simulink model "VanDerPol"  (R2015b)
settings: Solver=ode4  StartTime=0.0  StopTime=30  FixedStep=0.01  RelTol=1e-3
InitFcn:
  | clear all; close all; clc;
  | mu=1;
  | x0=1;
  | xdot0=0;
  | StartTime=0;
  | EndTime=26.7;
  | 
  | % Design LQR for NO feedforward
  | A=[1 -1;1 0]; B=[-1;0]; C=[0 1]; D=[0]; Q=[1 0;0 1];  R=[1]
  | [K,S,E] = lqr(A,B,Q,R)
  | 
  | Kp=K(1);  Kd=K(2);  Ki=Kp*0.1;
  | Kpo=1;  Kdo=Kpo*1;  Kio=Kpo*0;
StopFcn:
  | figure(1);
  | subplot(3,1,1); plot(t,Trajectory(:,1),'--r','linewidth',3); grid; ylabel('x(t)','fontsize',16); title('Position, Rate, Acceleration Trajectories','fontsize',16);
  | hold on; plot(t,State(:,1),'linewidth',2); hold off; legend('Desired', 'Actual');
  | subplot(3,1,2); plot(t,Trajectory(:,2),'--r','linewidth',3);  grid; ylabel('xdot(t)','fontsize',16);
  | hold on; plot(t,State(:,2),'linewidth',2);  hold off; legend('Desired', 'Actual');
  | subplot(3,1,3); plot(t,Trajectory(:,3),'--r','linewidth',3);  grid; ylabel('xddot(t)','fontsize',16); xlabel('time (sec)','fontsize',16);
  | hold on; plot(t,State(:,3),'linewidth',2);  hold off; legend('Desired', 'Actual');
  | 
  | MeanErrorX=num2str(mean(Trajectory(:,1)-State(:,1))); MeanErrorXdot=num2str(mean(Trajectory(:,2)-State(:,2)));MeanErrorXddot=num2str(mean(Trajectory(:,1)-State(:,3)));
  | STDErrorX=num2str(std(Trajectory(:,1)-State(:,1))); STDErrorXdot=num2str(std(Trajectory(:,2)-State(:,2)));STDErrorXddot=num2str(std(Trajectory(:,1)-State(:,3)));
  | ErrorLabelX=['\mu =',MeanErrorX, ',  \sigma= ',STDErrorX];  ErrorLabelXdot=['\mu =',MeanErrorXdot, ',  \sigma= ',STDErrorXdot];  ErrorLabelXddot=['\mu =',MeanErrorXddot, ',  \sigma= ',STDErrorXddot];
  | 
  | figure(2)
  | subplot(3,1,1); plot(t,Trajectory(:,1)-State(:,1),'linewidth',2); axis tight; grid; ylabel('\delta_x_(_t_)','fontsize',16);
  | title('ERROR: Position, Rate, Acceleration Trajectories','fontsize',16);   legend(ErrorLabelX);
  | 
  | subplot(3,1,2); plot(t,Trajectory(:,2)-State(:,2),'linewidth',2); axis tight; grid; ylabel('\delta_x_d_o_t_(_t_)','fontsize',16);
  | legend(ErrorLabelXdot);
  | 
  | subplot(3,1,3); plot(t,Trajectory(:,3)-State(:,3),'linewidth',2); axis tight; grid; ylabel('\delta_x_d_d_o_t_(_t_)','fontsize',16);
  | xlabel('time (sec)','fontsize',16);  legend(ErrorLabelXddot);
  | 
  | figure(3)
  | subplot(2,1,1); plot(t,LuenbergerEstimationError(:,1),'linewidth',2); axis tight; grid; ylabel('Luenberger','fontsize',16); title('Estimation \delta_x_(_t_) Error','fontsize',16);
  | subplot(2,1,2); plot(t,PIDoEstimationError,'linewidth',2); axis tight; grid; ylabel('PID','fontsize',16);
  | 
  | figure(4);plot(State(:,1), State(:,2)); axis equal; grid;
  | xlabel('x(t)','fontsize',16);; ylabel('dx(t)/dt','fontsize',16); title('Phase Portrait','fontsize',16);
libraries: simulink_need_slupdate x1, simulink x1
settings Model: Creator=tsands  LastModifiedBy=tasands
settings DataIOCC: SaveFormat=Array
settings DebuggingCC: UnderspecifiedInitializationDetection=Classic  MergeDetectMultiDrivingBlocksExec=none  SolverPrmCheckMsg=warning
settings HardwareCC: ProdBitPerPointer=32  ProdLargestAtomicFloat=None  ProdIntDivRoundTo=Undefined  ProdEndianess=Unspecified  ProdWordSize=32  ProdHWDeviceType=32-bit Generic
settings GRTTargetCC: GeneratePreprocessorConditionals=Disable all
settings ConfigComp: CovModelRefEnable=Off

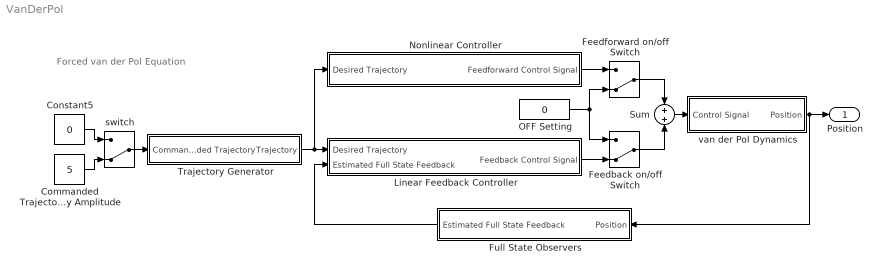
== system VanDerPol ==
  note: Forced van der Pol Equation
  " switch" : ManualSwitch  CurrentSetting=0
  Commanded Trajectory Amplitude : Constant  Value=5
  Constant5 : Constant  Value=0
  Feedback on/off Switch : ManualSwitch  CurrentSetting=0
  Feedforward on/off Switch : ManualSwitch  CurrentSetting=0
  Full State Observers : Subsystem
  Linear Feedback Controller : Subsystem
  Nonlinear Controller : Subsystem
  OFF Setting : Constant  Value=0
  Sum : Sum
  Trajectory Generator : Subsystem
  van der Pol Dynamics : Subsystem
  Position : Outport
  wires:
  van der Pol Dynamics/1(Position) -> Position/1, Full State Observers/1(Position)
  Sum/1 -> van der Pol Dynamics/1(Control Signal)
  Trajectory Generator/1(Trajectory) -> Nonlinear Controller/1(Desired Trajectory), Linear Feedback Controller/1(Desired Trajectory)
  Full State Observers/1(Estimated Full State Feedback) -> Linear Feedback Controller/2(Estimated Full State Feedback)
  Constant5/1 -> " switch"/1
  " switch"/1 -> Trajectory Generator/1(Commanded Trajectory)
  Commanded Trajectory Amplitude/1 -> " switch"/2
  OFF Setting/1 -> Feedforward on/off Switch/2, Feedback on/off Switch/1
  Nonlinear Controller/1(Feedforward Control Signal) -> Feedforward on/off Switch/1
  Feedforward on/off Switch/1 -> Sum/1
  Linear Feedback Controller/1(Feedback Control Signal) -> Feedback on/off Switch/2
  Feedback on/off Switch/1 -> Sum/2

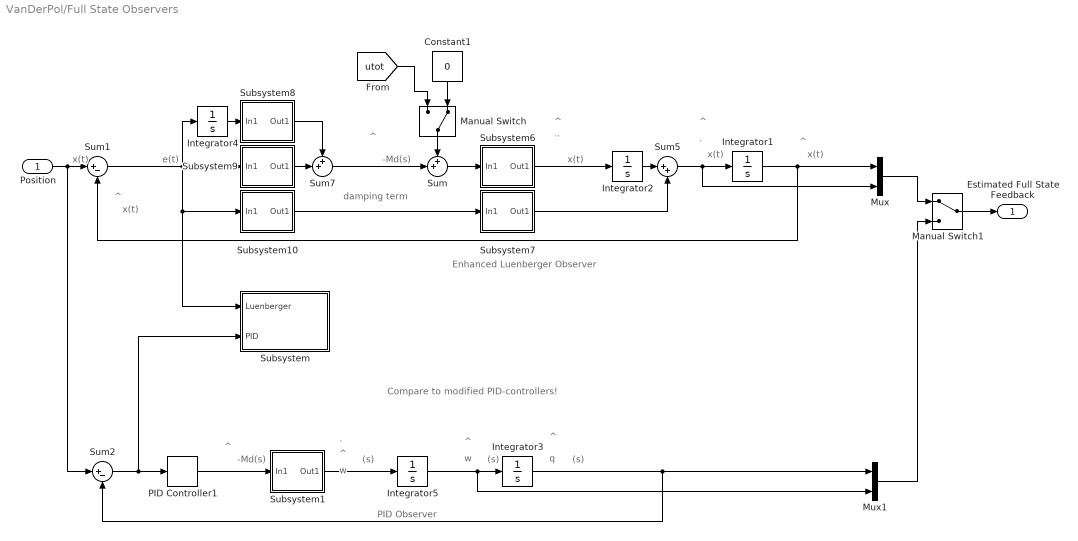
== system VanDerPol/Full State Observers ==
  note: PID Observer
  note: -Md(s)
  note: ^
  note: ^
  note: (s)
  note: w
  note: (s)
  note: .
  note: ^
  note: w
  note: e(t)
  note: damping term
  note: Enhanced Luenberger Observer
  note: ^
  note: x(t)
  note: x(t)
  note: ..
  note: ^
  note: x(t)
  note: ^
  note: ^
  note: -Md(s)
  note: (s)
  note: ^
  note: q
  note: Compare to modified PID-controllers!
  note: .
  note: x(t)
  note: ^
  note: x(t)
  Position : Inport
  Constant1 : Constant  Value=0
  Integrator{1..5} (5 alike) : Integrator
  Manual Switch : ManualSwitch  CurrentSetting=0
  Manual Switch1 : ManualSwitch
  Mux : Mux  Inputs=2
  Mux1 : Mux  Inputs=2
  PID Controller1 : simulink_need_slupdate/PID Controller  P=Kpo  I=Kio  D=Kdo
  Subsystem : Subsystem
      mask Display: disp('Scopes')
  Subsystem1 : Subsystem
      mask Display: disp('1/J^p')
  Subsystem10 : Subsystem
      mask Display: disp('Kdo')
  Subsystem6 : Subsystem
      mask Display: disp('1/J^p')
  Subsystem7 : Subsystem
      mask Display: disp('1/J^p')
  Subsystem8 : Subsystem
      mask Display: disp('Kio')
  Subsystem9 : Subsystem
      mask Display: disp('Kpo')
  Sum : Sum  Inputs=++|
  Sum1 : Sum  Inputs=|+-
  Sum2 : Sum  Inputs=|+-
  Sum5 : Sum  Inputs=|++
  Sum7 : Sum  Inputs=++|
  Estimated Full State Feedback : Outport
  wires:
  Manual Switch1/1 -> Estimated Full State Feedback/1
  Mux1/1 -> Manual Switch1/2
  Mux/1 -> Manual Switch1/1
  PID Controller1/1 -> Subsystem1/1(In1)
  Integrator3/1 -> Mux1/1, Sum2/2
  Integrator5/1 -> Mux1/2, Integrator3/1
  Subsystem1/1(Out1) -> Integrator5/1
  Manual Switch/1 -> Sum/1
  Constant1/1 -> Manual Switch/2
  [utot] -> Manual Switch/1
  Position/1 -> Sum1/1, Sum2/1
  Sum1/1 -> Subsystem/1(Luenberger), Subsystem10/1(In1), Subsystem9/1(In1), Integrator4/1
  Sum/1 -> Subsystem6/1(In1)
  Sum7/1 -> Sum/2
  Sum5/1 -> Mux/2, Integrator1/1
  Integrator4/1 -> Subsystem8/1(In1)
  Subsystem10/1(Out1) -> Subsystem7/1(In1)
  Subsystem9/1(Out1) -> Sum7/2
  Subsystem8/1(Out1) -> Sum7/1
  Subsystem7/1(Out1) -> Sum5/2
  Integrator2/1 -> Sum5/1
  Subsystem6/1(Out1) -> Integrator2/1
  Sum2/1 -> Subsystem/2(PID), PID Controller1/1
  Integrator1/1 -> Sum1/2, Mux/1

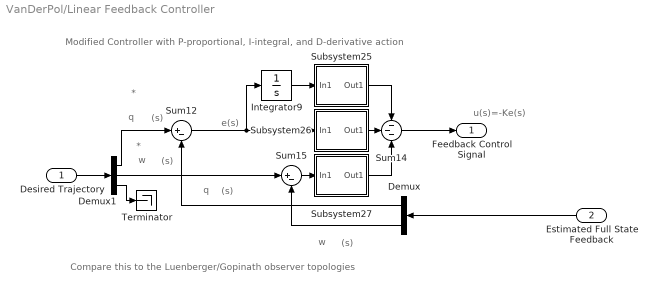
== system VanDerPol/Linear Feedback Controller ==
  note: e(s)
  note: w
  note: (s)
  note: q
  note: (s)
  note: u(s)=-Ke(s)
  note: *
  note: q
  note: (s)
  note: w
  note: *
  note: (s)
  note: Modified Controller with P-proportional, I-integral, and D-derivative action
  note: Compare this to the Luenberger/Gopinath observer topologies
  Desired Trajectory : Inport
  Estimated Full State Feedback : Inport  Port=2
  Demux : Demux  Outputs=2
  Demux1 : Demux  Outputs=3
  Integrator9 : Integrator
  Subsystem25 : Subsystem
      mask Display: disp('Ki')
  Subsystem26 : Subsystem
      mask Display: disp('Kp')
  Subsystem27 : Subsystem
      mask Display: disp('Kd')
  Sum12 : Sum  Inputs=|+-
  Sum14 : Sum  Inputs=---
  Sum15 : Sum  Inputs=|+-
  Terminator : Terminator
  Feedback Control Signal : Outport
  wires:
  Demux/1 -> Sum12/2
  Sum15/1 -> Subsystem27/1(In1)
  Integrator9/1 -> Subsystem25/1(In1)
  Sum12/1 -> Subsystem26/1(In1), Integrator9/1
  Subsystem27/1(Out1) -> Sum14/3
  Subsystem26/1(Out1) -> Sum14/2
  Subsystem25/1(Out1) -> Sum14/1
  Demux1/2 -> Sum15/1
  Demux1/1 -> Sum12/1
  Estimated Full State Feedback/1 -> Demux/1
  Demux/2 -> Sum15/2
  Desired Trajectory/1 -> Demux1/1
  Demux1/3 -> Terminator/1
  Sum14/1 -> Feedback Control Signal/1

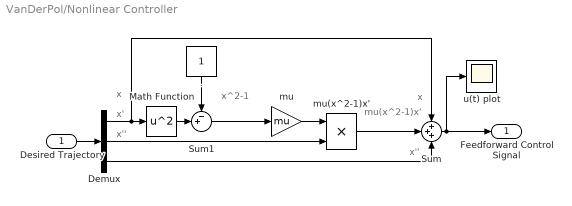
== system VanDerPol/Nonlinear Controller ==
  note: x
  note: x''
  note: mu(x^2-1)x'
  note: x''
  note: x'
  note: x
  note: x^2-1
  Desired Trajectory : Inport
  . : Constant
  Demux : Demux  Outputs=3
  Math Function : Math  Operator=square  SaturateOnIntegerOverflow=on
  Sum : Sum  Inputs=+++
  Sum1 : Sum  Inputs=-+|
  mu : Gain  Gain=mu
  mu(x^2-1)x' : Product
  u(t) plot : Scope
  Feedforward Control Signal : Outport
  wires:
  Desired Trajectory/1 -> Demux/1
  ./1 -> Sum1/1
  Math Function/1 -> Sum1/2
  Sum1/1 -> mu/1
  mu/1 -> mu(x^2-1)x'/1
  Demux/2 -> mu(x^2-1)x'/2
  mu(x^2-1)x'/1 -> Sum/2
  Demux/1 -> Sum/1, Math Function/1
  Demux/3 -> Sum/3
  Sum/1 -> Feedforward Control Signal/1, u(t) plot/1

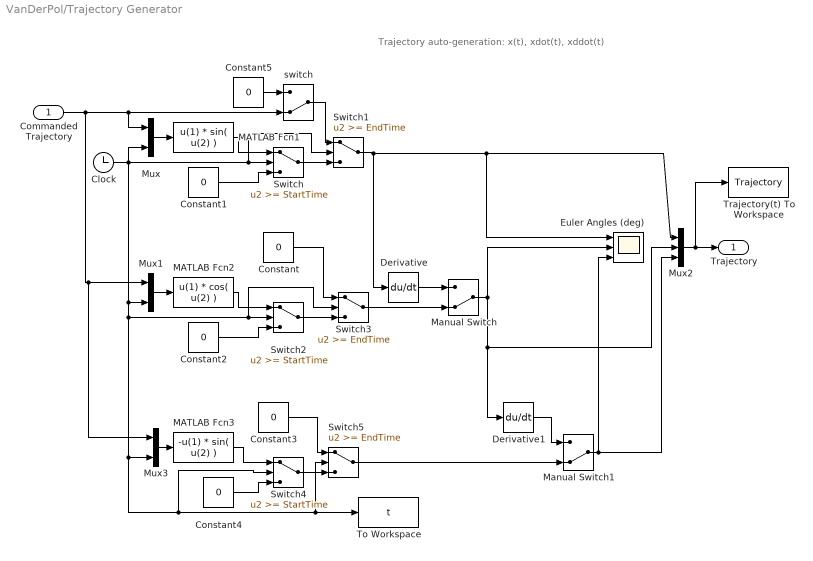
== system VanDerPol/Trajectory Generator ==
  note: Trajectory auto-generation: x(t), xdot(t), xddot(t)
  Commanded Trajectory : Inport
  " switch" : ManualSwitch  CurrentSetting=0
  Clock : Clock
  Constant{,1..5} (6 alike) : Constant  Value=0
  Derivative : Derivative
  Derivative1 : Derivative
  Euler Angles (deg) : Scope  NumInputPorts=3
      settings: StopFcn=|
      | %Simulink figure properties
      | shh=get(0,'ShowHiddenHandles');
      | set(0,'ShowHiddenHandles','On')
      | set(gcf,'menubar','figure')
      | set(gcf,'CloseRequestFcn','closereq')
      | set(gcf,'DefaultLineClipping','Off')
      | set(0,'ShowHiddenHandles',shh)
  MATLAB Fcn1 : MATLABFcn  MATLABFcn=u(1) * sin( u(2) )
  MATLAB Fcn2 : MATLABFcn  MATLABFcn=u(1) * cos( u(2) )
  MATLAB Fcn3 : MATLABFcn  MATLABFcn=-u(1) * sin( u(2) )
  Manual Switch : ManualSwitch  CurrentSetting=0
  Manual Switch1 : ManualSwitch  CurrentSetting=0
  Mux : Mux  Inputs=2
  Mux1 : Mux  Inputs=2
  Mux2 : Mux  Inputs=3
  Mux3 : Mux  Inputs=2
  Switch : Switch  Threshold=StartTime
  Switch1 : Switch  Threshold=EndTime
  Switch2 : Switch  Threshold=StartTime
  Switch3 : Switch  Threshold=EndTime
  Switch4 : Switch  Threshold=StartTime
  Switch5 : Switch  Threshold=EndTime
  To Workspace : ToWorkspace  VariableName=t  SampleTime=-1
  Trajectory(t) To Workspace : ToWorkspace  VariableName=Trajectory  SampleTime=-1
  Trajectory : Outport
  wires:
  Mux2/1 -> Trajectory(t) To Workspace/1, Trajectory/1
  Switch1/1 -> Mux2/1, Euler Angles (deg)/1, Derivative/1
  Switch5/1 -> Manual Switch1/2
  Derivative1/1 -> Manual Switch1/1
  Switch3/1 -> Manual Switch/2
  Derivative/1 -> Manual Switch/1
  MATLAB Fcn3/1 -> Switch4/1
  Switch/1 -> Switch1/3
  Constant1/1 -> Switch/3
  MATLAB Fcn1/1 -> Switch/1
  Commanded Trajectory/1 -> " switch"/2, Mux/1, Mux3/1, Mux1/1
  Mux/1 -> MATLAB Fcn1/1
  Manual Switch/1 -> Mux2/2, Derivative1/1, Euler Angles (deg)/2
  Mux1/1 -> MATLAB Fcn2/1
  MATLAB Fcn2/1 -> Switch2/1
  Constant2/1 -> Switch2/3
  Switch2/1 -> Switch3/3
  Constant/1 -> Switch3/1
  Constant3/1 -> Switch5/1
  Switch4/1 -> Switch5/3
  Constant4/1 -> Switch4/3
  Manual Switch1/1 -> Mux2/3, Euler Angles (deg)/3
  Clock/1 -> Switch/2, Switch1/2, Mux/2, Mux1/2, Switch3/2, Switch2/2, Switch4/2, Switch5/2, To Workspace/1, Mux3/2
  Mux3/1 -> MATLAB Fcn3/1
  Constant5/1 -> " switch"/1
  " switch"/1 -> Switch1/1

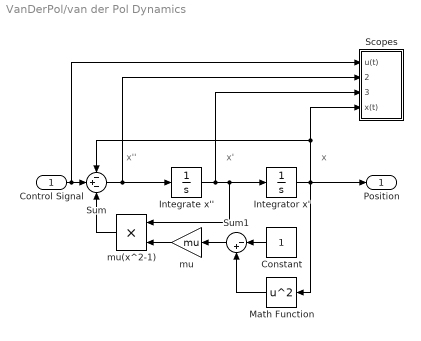
== system VanDerPol/van der Pol Dynamics ==
  note: x''
  note: x'
  note: x
  Control Signal : Inport
  Constant : Constant
  Integrate x'' : Integrator  InitialCondition=xdot0
  Integrator x' : Integrator  InitialCondition=x0
  Math Function : Math  Operator=square  SaturateOnIntegerOverflow=on
  Scopes : Subsystem
  Sum : Sum  Inputs=-+-
  Sum1 : Sum  Inputs=|-+
  mu : Gain  Gain=mu
  mu(x^2-1) : Product
  Position : Outport
  wires:
  mu(x^2-1)/1 -> Sum/3
  Control Signal/1 -> Scopes/1(u(t)), Sum/2
  Constant/1 -> Sum1/1
  Math Function/1 -> Sum1/2
  mu/1 -> mu(x^2-1)/2
  Integrator x'/1 -> Sum/1, Scopes/4(x(t)), Math Function/1, Position/1
  Sum1/1 -> mu/1
  Sum/1 -> Scopes/2(xddot(t)), Integrate x''/1
  Integrate x''/1 -> Integrator x'/1, mu(x^2-1)/1, Scopes/3(xdot(t))

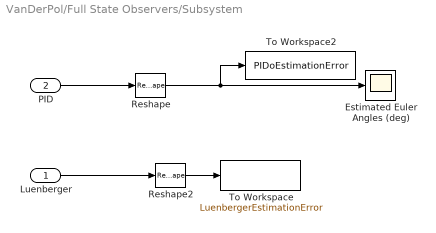
== system VanDerPol/Full State Observers/Subsystem ==
  Luenberger : Inport
  PID : Inport  Port=2
  Estimated Euler Angles (deg) : Scope
      settings: StopFcn=|
      | %Simulink figure properties
      | shh=get(0,'ShowHiddenHandles');
      | set(0,'ShowHiddenHandles','On')
      | set(gcf,'menubar','figure')
      | set(gcf,'CloseRequestFcn','closereq')
      | set(gcf,'DefaultLineClipping','Off')
      | set(0,'ShowHiddenHandles',shh)
  Reshape : Reshape
  Reshape2 : Reshape  OutputDimensions=[1,9]
  To Workspace : ToWorkspace  VariableName=LuenbergerEstimationError  SampleTime=-1
  To Workspace2 : ToWorkspace  VariableName=PIDoEstimationError  SampleTime=-1
  wires:
  PID/1 -> Reshape/1
  Reshape/1 -> To Workspace2/1, Estimated Euler Angles (deg)/1
  Reshape2/1 -> To Workspace/1
  Luenberger/1 -> Reshape2/1

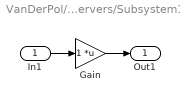
== system VanDerPol/Full State Observers/Subsystem1 ==
  In1 : Inport
  Gain : Gain  Multiplication=Matrix(K*u)
  Out1 : Outport
  wires:
  In1/1 -> Gain/1
  Gain/1 -> Out1/1

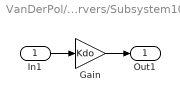
== system VanDerPol/Full State Observers/Subsystem10 ==
  In1 : Inport
  Gain : Gain  Gain=Kdo
  Out1 : Outport
  wires:
  Gain/1 -> Out1/1
  In1/1 -> Gain/1

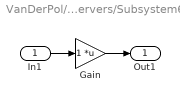
== system VanDerPol/Full State Observers/Subsystem6 ==
  In1 : Inport
  Gain : Gain  Multiplication=Matrix(K*u)
  Out1 : Outport
  wires:
  Gain/1 -> Out1/1
  In1/1 -> Gain/1

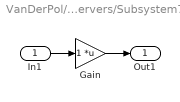
== system VanDerPol/Full State Observers/Subsystem7 ==
  In1 : Inport
  Gain : Gain  Multiplication=Matrix(K*u)
  Out1 : Outport
  wires:
  In1/1 -> Gain/1
  Gain/1 -> Out1/1

== system VanDerPol/Full State Observers/Subsystem8 ==
  In1 : Inport
  Gain : Gain  Gain=Kio
  Out1 : Outport
  wires:
  Gain/1 -> Out1/1
  In1/1 -> Gain/1

== system VanDerPol/Full State Observers/Subsystem9 ==
  In1 : Inport
  Gain : Gain  Gain=Kpo
  Out1 : Outport
  wires:
  In1/1 -> Gain/1
  Gain/1 -> Out1/1

== system VanDerPol/Linear Feedback Controller/Subsystem25 ==
  In1 : Inport
  Ki : Gain  Gain=Ki
  Out1 : Outport
  wires:
  In1/1 -> Ki/1
  Ki/1 -> Out1/1

== system VanDerPol/Linear Feedback Controller/Subsystem26 ==
  In1 : Inport
  Gain : Gain  Gain=Kp
  Out1 : Outport
  wires:
  Gain/1 -> Out1/1
  In1/1 -> Gain/1

== system VanDerPol/Linear Feedback Controller/Subsystem27 ==
  In1 : Inport
  Gain : Gain  Gain=Kd
  Out1 : Outport
  wires:
  In1/1 -> Gain/1
  Gain/1 -> Out1/1

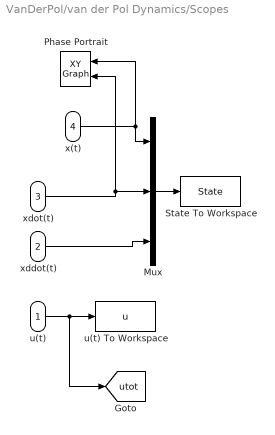
== system VanDerPol/van der Pol Dynamics/Scopes ==
  u(t) : Inport
  xddot(t) : Inport  Port=2
  xdot(t) : Inport  Port=3
  x(t) : Inport  Port=4
  Mux : Mux  Inputs=3
  Phase Portrait : simulink/Sinks/XY Graph  xmin=-10  xmax=10  ymin=-10  ymax=10  st=-1
  State To Workspace : ToWorkspace  VariableName=State  SampleTime=-1
  u(t) To Workspace : ToWorkspace  VariableName=u  SampleTime=-1
  tag scope: utot=global
  wires:
  u(t)/1 -> [utot], u(t) To Workspace/1
  x(t)/1 -> Mux/1, Phase Portrait/1
  xdot(t)/1 -> Phase Portrait/2, Mux/2
  xddot(t)/1 -> Mux/3
  Mux/1 -> State To Workspace/1
